simulink model "Channelizer"  (R2026a)
settings: Solver=VariableStepAuto  StopTime=1e-5
InitFcn:
  | init;
values from neighbouring files (symbols this model uses):
  ch0_en = 0    [channelizer_demo_init.m]    (also in init.m)
  ch0_qam = 0    [channelizer_demo_init.m]    (also in init.m)
  ch0_swp = 0    [channelizer_demo_init.m]    (also in init.m)
  ch10_en = 0    [channelizer_demo_init.m]    (also in init.m)
  ch10_qam = 0    [channelizer_demo_init.m]    (also in init.m)
  ch10_swp = 0    [channelizer_demo_init.m]    (also in init.m)
  ch11_en = 0    [channelizer_demo_init.m]    (also in init.m)
  ch11_qam = 0    [channelizer_demo_init.m]    (also in init.m)
  ch11_swp = 0    [channelizer_demo_init.m]    (also in init.m)
  ch12_en = 0    [channelizer_demo_init.m]    (also in init.m)
  ch12_qam = 0    [channelizer_demo_init.m]    (also in init.m)
  ch12_swp = 0    [channelizer_demo_init.m]    (also in init.m)
  ch13_en = 0    [channelizer_demo_init.m]    (also in init.m)
  ch13_qam = 0    [channelizer_demo_init.m]    (also in init.m)
  ch13_swp = 0    [channelizer_demo_init.m]    (also in init.m)
  ch14_en = 0    [channelizer_demo_init.m]    (also in init.m)
  ch14_qam = 0    [channelizer_demo_init.m]    (also in init.m)
  ch14_swp = 0    [channelizer_demo_init.m]    (also in init.m)
  ch15_en = 0    [channelizer_demo_init.m]    (also in init.m)
  ch15_qam = 0    [channelizer_demo_init.m]    (also in init.m)
  ch15_swp = 0    [channelizer_demo_init.m]    (also in init.m)
  ch1_en = 1    [channelizer_demo_init.m]    (also in init.m)
  ch1_qam = 0    [channelizer_demo_init.m]    (also in init.m)
  ch1_swp = 0    [channelizer_demo_init.m]    (also in init.m)
  ch2_en = 1    [channelizer_demo_init.m]    (also in init.m)
  ch2_qam = 0    [channelizer_demo_init.m]    (also in init.m)
  ch2_swp = 0    [channelizer_demo_init.m]    (also in init.m)
  ch3_en = 0    [channelizer_demo_init.m]    (also in init.m)
  ch3_qam = 0    [channelizer_demo_init.m]    (also in init.m)
  ch3_swp = 0    [channelizer_demo_init.m]    (also in init.m)
  ch4_en = 0    [channelizer_demo_init.m]    (also in init.m)
  ch4_qam = 0    [channelizer_demo_init.m]    (also in init.m)
  ch4_swp = 0    [channelizer_demo_init.m]    (also in init.m)
  ch5_en = 1    [channelizer_demo_init.m]    (also in init.m)
  ch5_qam = 1    [channelizer_demo_init.m]    (also in init.m)
  ch5_swp = 0    [channelizer_demo_init.m]    (also in init.m)
  ch6_en = 1    [channelizer_demo_init.m]    (also in init.m)
  ch6_qam = 1    [channelizer_demo_init.m]    (also in init.m)
  ch6_swp = 0    [channelizer_demo_init.m]    (also in init.m)
  ch7_en = 0    [channelizer_demo_init.m]    (also in init.m)
  ch7_qam = 0    [channelizer_demo_init.m]    (also in init.m)
  ch7_swp = 0    [channelizer_demo_init.m]    (also in init.m)
  ch8_en = 0    [channelizer_demo_init.m]    (also in init.m)
  ch8_qam = 0    [channelizer_demo_init.m]    (also in init.m)
  ch8_swp = 0    [channelizer_demo_init.m]    (also in init.m)
  ch9_en = 0    [channelizer_demo_init.m]    (also in init.m)
  ch9_qam = 0    [channelizer_demo_init.m]    (also in init.m)
  ch9_swp = 0    [channelizer_demo_init.m]    (also in init.m)
  ch_filt_coef = 28 * ch_filt_coef / sum(ch_filt_coef(:))    [init.m]
  N = 2*1024    (= 2048)    [hil.m]    (also in init.m = 256)
  nvar = 0.01    [init.m]
  randph = 2*pi*rand(16,1)    [init.m]
  spec1_ch = 1    [channelizer_demo_init.m]    (also in init.m)
  spec2_ch = 2    [channelizer_demo_init.m]    (also in init.m)
  spec3_ch = 5    [channelizer_demo_init.m]    (also in init.m)
  spec4_ch = 6    [channelizer_demo_init.m]    (also in init.m)
  swp_rate0 = 0    [channelizer_demo_init.m]    (also in init.m)
  swp_rate1 = 0    [channelizer_demo_init.m]    (also in init.m)
  swp_rate10 = 0    [channelizer_demo_init.m]    (also in init.m)
  swp_rate11 = 0    [channelizer_demo_init.m]    (also in init.m)
  swp_rate12 = 0    [channelizer_demo_init.m]    (also in init.m)
  swp_rate13 = 0    [channelizer_demo_init.m]    (also in init.m)
  swp_rate14 = 0    [channelizer_demo_init.m]    (also in init.m)
  swp_rate15 = 0    [channelizer_demo_init.m]    (also in init.m)
  swp_rate2 = 0    [channelizer_demo_init.m]    (also in init.m)
  swp_rate3 = 0    [channelizer_demo_init.m]    (also in init.m)
  swp_rate4 = 0    [channelizer_demo_init.m]    (also in init.m)
  swp_rate5 = 0    [channelizer_demo_init.m]    (also in init.m)
  swp_rate6 = 0    [channelizer_demo_init.m]    (also in init.m)
  swp_rate7 = 0    [channelizer_demo_init.m]    (also in init.m)
  swp_rate8 = 0    [channelizer_demo_init.m]    (also in init.m)
  swp_rate9 = 0    [channelizer_demo_init.m]    (also in init.m)
  Ts = 16*(7/4)/8.75e9    (= 3.2e-09)    [init.m]
undefined symbols (not defined in the file or in its folder): Asymmetric, jsin, S, vsva2197, xcvc1902
libraries: aieUtilities x20, aieBasic x7, hlsBasic x4, aieDSP x2, vmcUtilities x1
(part 1 of 3)
settings Model: Creator=robg  LastModifiedBy=robg
settings DebuggingCC: ParameterOverflowMsg=none  ParameterPrecisionLossMsg=none

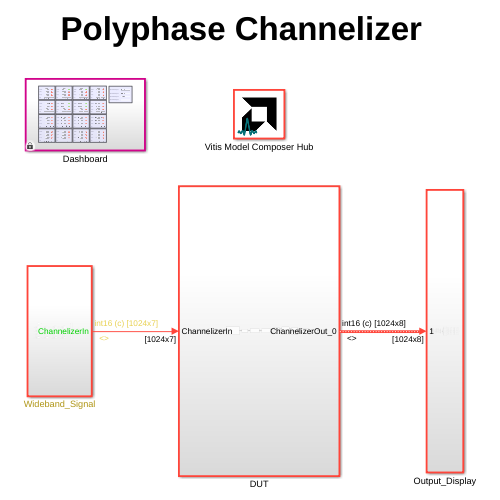
[thumbnail: Simulink's stored preview of the top-level diagram]
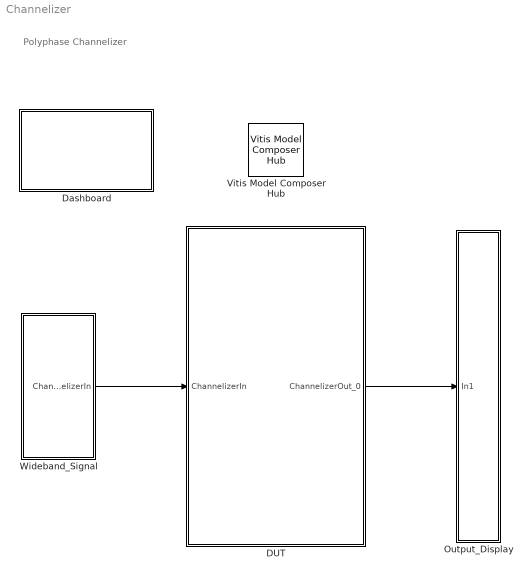
== system Channelizer ==
  note: Polyphase Channelizer
  DUT : Subsystem
  Dashboard : Subsystem
  Output_Display : Subsystem
  Vitis Model Composer Hub : vmcUtilities/Vitis Model Composer Hub  Tag=genX  CodeGeneration=off  SubsystemName=AIE_DFT_SSR  BlockHierPath=Channelizer/DUT/AIE_DFT_SSR  CompilationType=AIECompilation  SubsystemType=AIENode  AIEArrayConfig=Use entire AIE array  StartColumn=1  NumberOfColumns=1  TargetDirectory=./analyze_ssr4  exportDesign=off  analyzeDesign=on  validateDesignOnHw=off  ExportType=AI Engines  IpVendor=xilinx.com  IpLibrary=hls  IpVersion=1.0  IpHWLanguage=Verilog  AieCompilerOptions={}  AieSimulatorOptions={}  CreateTestbench=on  TestbenchStackSize=10  RunRtlSim=off  RunCSim=off  RunAieSim=on  enableSimulationTimeout=on  enableGraphIterations=on  AieSimTimeout=50000  AieGraphIterations=-1  RunAieSimProfiling=on  LaunchVitisAnalyzer=off  PlotOutput=off  RunX86Sim=off  X86SimTimeout=10  GenHwImage=off  GenLibadfXo=off  GenHwValidationCode=off  PlatformType=Not Specified  HwSystemType=Baremetal  HwValidationTarget=hw  ProjDevice=Versal VCK190 Evaluation Platform (xcvc1902-vsva2197-2MP-e-S)  ProjDevicePart=xcvc1902-vsva2197-2MP-e-S  AIEType=AIE  SamplePeriod=-1  ClockFrequency=200  DataPathParallelism=1  xilinxfamily=versalaicore  part=xcvc1902  speed=-2MP-e-S  package=vsva2197  directory=./netlist  testbench=off  incr_netlist=off  synthesis_tool=Vivado  clock_wrapper=Clock Enables  dbl_ovrd=According to Block Masks  dcm_input_clock_period=10  sysclk_period=10  simulink_period=1  eval_field=0  IPInfoJsonString="{\"DUTSubsystemName\":\"AIE_DFT_SSR\",\"AIESubsystem\":{\"SubsystemName\":\"AIE_DFT_SSR\",\"TargetDirectory\":\"./analyze_ssr4\",\"AIEArrayConfig\":\"Use entire AIE array\",\"StartColumn\":\"0\",\"NumberOfColumns\":\"1\"},\"SubsystemTag\":\"AIENode\"}"  LogFileName=/group/xcoswmktg2/robg/git/vmc/Vitis_Model_Composer/Examples/AIENGINE_plus_PL/AIE_HLS/Channelizer/code_dut_ssr_vss/model_composer.log  NThreads=4  IPConfigFile=/tmp/vmctmp-12614866774650903480/Channelizer_ipconfig.json
  Wideband_Signal : Subsystem
  wires:
  DUT/1(ChannelizerOut_0) -> Output_Display/1(In1)
  Wideband_Signal/1(ChannelizerIn) -> DUT/1(ChannelizerIn)

== system Channelizer/DUT ==
  ChannelizerIn : Inport
  AIE to HLS15 : aieUtilities/AIE to HLS  OutputType=ufix128  OutputSize=N  AllowMultiRate=off  InputType=int8
  AIE to HLS16 : aieUtilities/AIE to HLS  OutputType=ufix128  OutputSize=N  AllowMultiRate=off  InputType=int8
  AIE_DFT_SSR : Subsystem
  AIE_FilterBank_SSR : Subsystem
  AIE_to_HLS_IDFT_Out_0 : aieUtilities/AIE to HLS  OutputType=ufix128  OutputSize=1024  AllowMultiRate=off  InputType=cint16
  AIE_to_HLS_IDFT_Out_1 : aieUtilities/AIE to HLS  OutputType=ufix128  OutputSize=1024  AllowMultiRate=off  InputType=cint16
  HLS to AIE17 : aieUtilities/HLS to AIE  OutputType=cint16  OutputSize=4*N  AllowMultiRate=off  InputType=cint16
  HLS_to_AIE_Channel_0 : aieUtilities/HLS to AIE  OutputType=cint16  OutputSize=1024  AllowMultiRate=off  InputType=cint16
  HLS_to_AIE_IDFT_Half0 : aieUtilities/HLS to AIE  OutputType=cint16  OutputSize=2048  AllowMultiRate=off  InputType=cint16
  HLS_to_AIE_IDFT_Half1 : aieUtilities/HLS to AIE  OutputType=cint16  OutputSize=2048  AllowMultiRate=off  InputType=cint16
  idft_output_unpack_kernel : hlsBasic/HLS Kernel  PortNames={'return'; 'half0'; 'half1'; 'hops'}  PortSerializedTypes={'{Bv}';'{C{Thls::stream{2{t{Tap_uint{1{t{}128}}}}{t{}0}}}4}';'{C{Thls::stream{2{t{Tap_uint{1{t{}128}}}}{t{}0}}}4}';'{C{Thls::stream{2{t{Tap_uint{1{t{}128}}}}{t{}0}}}8}'}  FunctionTemplateSpecKind=none  FunctionTemplateParamNames={}  FunctionTemplateParamKinds={}  FunctionTemplateParamTypes={}  FunctionTemplateParamValues={}  PortSynchronicities={'auto'; 'auto'; 'auto'}  PortSignalSizes={0.000000000000000000e+00; 0.000000000000000000e+00; 2.560000000000000000e+02}  PortParameterValues={}  PortAttributesTable={'Input', 'half0', 'hls::stream< ap_uint< 128 >, 0 >[ 4 ]', '', '';'Input', 'half1', 'hls::stream< ap_uint< 128 >, 0 >[ 4 ]', '', '';'Output', 'hops', 'hls::stream< ap_uint< 128 >, 0 >[ 8 ]', '', '256'}  PortAttributesEnablement={'off', 'off', 'off', 'off', 'off';'off', 'off', 'off', 'off', 'off';'off', 'off', 'off', 'off', 'on'}  PortParametersTable={}  SampleTime=-1  PortDirectionTable={'half0', 'hls::stream< ap_uint< 128 >, 0 >[ 4 ]', 'Input', 'Port';'half1', 'hls::stream< ap_uint< 128 >, 0 >[ 4 ]', 'Input', 'Port';'hops', 'hls::stream< ap_uint< 128 >, 0 >[ 8 ]', 'Output', 'Port'}  FunctionTemplateParams={}  FunctionTemplateParamsEnables={}  FunctionTemplateParamsVisible=off  FunctionDeclTypeOptions=C[1 1]@t7@<empty>  PortDirectionTabVisible=on  ArgDirections={1.000000000000000000e+00; 1.000000000000000000e+00; 2.000000000000000000e+00}  ArgInterfaceTypes={1.000000000000000000e+00; 1.000000000000000000e+00; 1.000000000000000000e+00}  FunctionIndex=1  FormalArgDecls={'hls::stream< ap_uint< 128 >, 0 > half0 [ 4 ]';'hls::stream< ap_uint< 128 >, 0 > half1 [ 4 ]';'hls::stream< ap_uint< 128 >, 0 > hops [ 8 ]'}  SimLibPath=''  FunctionTabVisible=on  FunctionDescription=void idft_output_unpack_kernel(hls::stream< ap_uint< 128 >, 0 > half0 [ 4 ], hls::stream< ap_uint< 128 >, 0 > half1 [ 4 ], hls::stream< ap_uint< 128 >, 0 > hops [ 8 ])  blockJsonConstraints=[]  deprecateConstraints=0  KernelHeaderFile=hls/idft_output_unpack_ssr4.h  KernelFunction=idft_output_unpack_kernel  KernelFunctionSelect=<empty>  KernelSourceFile=hls/idft_output_unpack_ssr4.cpp  KernelSearchPaths={}  PreProcOptions={}
  m16_ssr8_cshift_idft_array : hlsBasic/HLS Kernel  PortNames={'return'; 'sig_i'; 'half0'; 'half1'}  PortSerializedTypes={'{Bv}';'{C{Thls::stream{2{t{Tap_uint{1{t{}128}}}}{t{}0}}}8}';'{C{Thls::stream{2{t{Tap_uint{1{t{}128}}}}{t{}0}}}16}';'{C{Thls::stream{2{t{Tap_uint{1{t{}128}}}}{t{}0}}}16}'}  FunctionTemplateSpecKind=none  FunctionTemplateParamNames={}  FunctionTemplateParamKinds={}  FunctionTemplateParamTypes={}  FunctionTemplateParamValues={}  PortSynchronicities={'auto'; 'auto'; 'auto'}  PortSignalSizes={0.000000000000000000e+00; 5.120000000000000000e+02; 5.120000000000000000e+02}  PortParameterValues={}  PortAttributesTable={'Input', 'sig_i', 'hls::stream< ap_uint< 128 >, 0 >[ 8 ]', '', '';'Output', 'half0', 'hls::stream< ap_uint< 128 >, 0 >[ 16 ]', '', '512';'Output', 'half1', 'hls::stream< ap_uint< 128 >, 0 >[ 16 ]', '', '512'}  PortAttributesEnablement={'off', 'off', 'off', 'off', 'off';'off', 'off', 'off', 'off', 'on';'off', 'off', 'off', 'off', 'on'}  PortParametersTable={}  SampleTime=-1  PortDirectionTable={'sig_i', 'hls::stream< ap_uint< 128 >, 0 >[ 8 ]', 'Input', 'Port';'half0', 'hls::stream< ap_uint< 128 >, 0 >[ 16 ]', 'Output', 'Port';'half1', 'hls::stream< ap_uint< 128 >, 0 >[ 16 ]', 'Output', 'Port'}  FunctionTemplateParams={}  FunctionTemplateParamsEnables={}  FunctionTemplateParamsVisible=off  FunctionDeclTypeOptions=C[1 1]@t7@<empty>  PortDirectionTabVisible=on  ArgDirections={1.000000000000000000e+00; 2.000000000000000000e+00; 2.000000000000000000e+00}  ArgInterfaceTypes={1.000000000000000000e+00; 1.000000000000000000e+00; 1.000000000000000000e+00}  FunctionIndex=1  FormalArgDecls={'hls::stream< ap_uint< 128 >, 0 > sig_i [ 8 ]';'hls::stream< ap_uint< 128 >, 0 > half0 [ 16 ]';'hls::stream< ap_uint< 128 >, 0 > half1 [ 16 ]'}  SimLibPath=''  FunctionTabVisible=on  FunctionDescription=void m16_ssr8_cshift_idft_array(hls::stream< ap_uint< 128 >, 0 > sig_i [ 8 ], hls::stream< ap_uint< 128 >, 0 > half0 [ 16 ], hls::stream< ap_uint< 128 >, 0 > half1 [ 16 ])  blockJsonConstraints=[]  deprecateConstraints=0  KernelHeaderFile=hls/m16_ssr8_cyclic_shift_ssr4.h  KernelFunction=m16_ssr8_cshift_idft_array  KernelFunctionSelect=<empty>  KernelSourceFile=hls/m16_ssr8_cyclic_shift_ssr4.cpp  KernelSearchPaths={}  PreProcOptions={}
  m16_ssr8_permute_fb_i_array : hlsBasic/HLS Kernel  PortNames={'return'; 'sig_i'; 'sig_o'}  PortSerializedTypes={'{Bv}'; '{C{Thls::stream{2{t{Tap_uint{1{t{}128}}}}{t{}0}}}7}'; '{C{Thls::stream{2{t{Tap_uint{1{t{}128}}}}{t{}0}}}8}'}  FunctionTemplateSpecKind=none  FunctionTemplateParamNames={}  FunctionTemplateParamKinds={}  FunctionTemplateParamTypes={}  FunctionTemplateParamValues={}  PortSynchronicities={'auto'; 'auto'}  PortSignalSizes={0.000000000000000000e+00; 2.560000000000000000e+02}  PortParameterValues={}  PortAttributesTable={ 'Input', 'sig_i', 'hls::stream< ap_uint< 128 >, 0 >[ 7 ]', '', ''; 'Output', 'sig_o', 'hls::stream< ap_uint< 128 >, 0 >[ 8 ]', '', 'N' }  PortAttributesEnablement={'off', 'off', 'off', 'off', 'off';'off', 'off', 'off', 'off', 'on'}  PortParametersTable={}  SampleTime=-1  PortDirectionTable={ 'sig_i', 'hls::stream< ap_uint< 128 >, 0 >[ 7 ]', 'Input', 'Port'; 'sig_o', 'hls::stream< ap_uint< 128 >, 0 >[ 8 ]', 'Output', 'Port' }  FunctionTemplateParams={}  FunctionTemplateParamsEnables={}  FunctionTemplateParamsVisible=off  FunctionDeclTypeOptions=C[1 1]@t7@<empty>  PortDirectionTabVisible=on  ArgDirections={1.000000000000000000e+00; 2.000000000000000000e+00}  ArgInterfaceTypes={1.000000000000000000e+00; 1.000000000000000000e+00}  FunctionIndex=1  FormalArgDecls={'hls::stream< ap_uint< 128 >, 0 > sig_i [ 7 ]', 'hls::stream< ap_uint< 128 >, 0 > sig_o [ 8 ]'}  SimLibPath=''  FunctionTabVisible=on  FunctionDescription=void m16_ssr8_permute_fb_i_array(hls::stream< ap_uint< 128 >, 0 > sig_i [ 7 ], hls::stream< ap_uint< 128 >, 0 > sig_o [ 8 ])  blockJsonConstraints=[]  deprecateConstraints=0  KernelHeaderFile=hls/m16_ssr8_permute_fb_i.h  KernelFunction=m16_ssr8_permute_fb_i_array  KernelFunctionSelect=<empty>  KernelSourceFile=hls/m16_ssr8_permute_fb_i.cpp  KernelSearchPaths={}  PreProcOptions={}
  m16_ssr8_permute_fb_o_array : hlsBasic/HLS Kernel  PortNames={'return'; 'sig_i'; 'sig_o'}  PortSerializedTypes={'{Bv}'; '{C{Thls::stream{2{t{Tap_uint{1{t{}128}}}}{t{}0}}}8}'; '{C{Thls::stream{2{t{Tap_uint{1{t{}128}}}}{t{}0}}}8}'}  FunctionTemplateSpecKind=none  FunctionTemplateParamNames={}  FunctionTemplateParamKinds={}  FunctionTemplateParamTypes={}  FunctionTemplateParamValues={}  PortSynchronicities={'auto'; 'auto'}  PortSignalSizes={0.000000000000000000e+00; 2.560000000000000000e+02}  PortParameterValues={}  PortAttributesTable={ 'Input', 'sig_i', 'hls::stream< ap_uint< 128 >, 0 >[ 8 ]', '', ''; 'Output', 'sig_o', 'hls::stream< ap_uint< 128 >, 0 >[ 8 ]', '', 'N' }  PortAttributesEnablement={'off', 'off', 'off', 'off', 'off';'off', 'off', 'off', 'off', 'on'}  PortParametersTable={}  SampleTime=-1  PortDirectionTable={ 'sig_i', 'hls::stream< ap_uint< 128 >, 0 >[ 8 ]', 'Input', 'Port'; 'sig_o', 'hls::stream< ap_uint< 128 >, 0 >[ 8 ]', 'Output', 'Port' }  FunctionTemplateParams={}  FunctionTemplateParamsEnables={}  FunctionTemplateParamsVisible=off  FunctionDeclTypeOptions=C[1 1]@t7@<empty>  PortDirectionTabVisible=on  ArgDirections={1.000000000000000000e+00; 2.000000000000000000e+00}  ArgInterfaceTypes={1.000000000000000000e+00; 1.000000000000000000e+00}  FunctionIndex=1  FormalArgDecls={'hls::stream< ap_uint< 128 >, 0 > sig_i [ 8 ]', 'hls::stream< ap_uint< 128 >, 0 > sig_o [ 8 ]'}  SimLibPath=''  FunctionTabVisible=on  FunctionDescription=void m16_ssr8_permute_fb_o_array(hls::stream< ap_uint< 128 >, 0 > sig_i [ 8 ], hls::stream< ap_uint< 128 >, 0 > sig_o [ 8 ])  blockJsonConstraints=[]  deprecateConstraints=0  KernelHeaderFile=hls/m16_ssr8_permute_fb_o.h  KernelFunction=m16_ssr8_permute_fb_o_array  KernelFunctionSelect=<empty>  KernelSourceFile=hls/m16_ssr8_permute_fb_o.cpp  KernelSearchPaths={}  PreProcOptions={}
  ChannelizerOut_0 : Outport
  wires:
  HLS_to_AIE_Channel_0/1 -> ChannelizerOut_0/1
  idft_output_unpack_kernel/1 -> HLS_to_AIE_Channel_0/1
  AIE_to_HLS_IDFT_Out_1/1 -> idft_output_unpack_kernel/2
  ChannelizerIn/1 -> AIE to HLS16/1
  AIE_to_HLS_IDFT_Out_0/1 -> idft_output_unpack_kernel/1
  AIE to HLS16/1 -> m16_ssr8_permute_fb_i_array/1
  AIE_FilterBank_SSR/1(Out1) -> AIE to HLS15/1
  AIE to HLS15/1 -> m16_ssr8_permute_fb_o_array/1
  HLS to AIE17/1 -> AIE_FilterBank_SSR/1(In1)
  HLS_to_AIE_IDFT_Half0/1 -> AIE_DFT_SSR/1(In_Half0)
  m16_ssr8_permute_fb_o_array/1 -> m16_ssr8_cshift_idft_array/1
  m16_ssr8_cshift_idft_array/1 -> HLS_to_AIE_IDFT_Half0/1
  m16_ssr8_cshift_idft_array/2 -> HLS_to_AIE_IDFT_Half1/1
  m16_ssr8_permute_fb_i_array/1 -> HLS to AIE17/1
  HLS_to_AIE_IDFT_Half1/1 -> AIE_DFT_SSR/2(In_Half1)
  AIE_DFT_SSR/1(IDFT_Half0_Out) -> AIE_to_HLS_IDFT_Out_0/1
  AIE_DFT_SSR/2(IDFT_Half1_Out) -> AIE_to_HLS_IDFT_Out_1/1

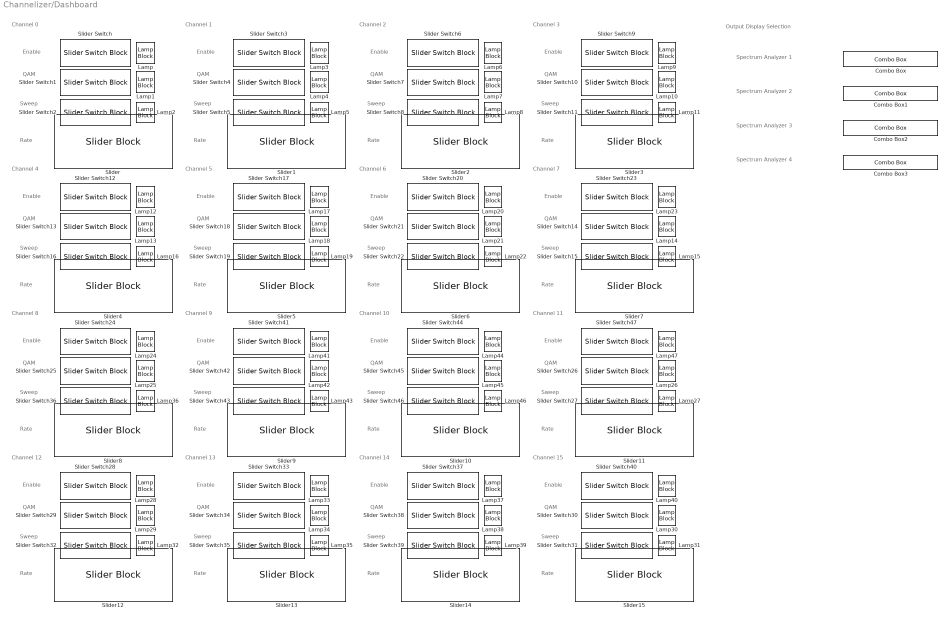
== system Channelizer/Dashboard ==
  note: Output Display Selection
  note: Spectrum Analyzer 1
  note: Enable
  note: Channel 0
  note: QAM
  note: Sweep
  note: Rate
  note: Channel 1
  note: Rate
  note: QAM
  note: Sweep
  note: Enable
  note: Channel 2
  note: Channel 3
  note: Rate
  note: Enable
  note: QAM
  note: Sweep
  note: QAM
  note: Sweep
  note: Rate
  note: Enable
  note: QAM
  note: Enable
  note: Rate
  note: Sweep
  note: Rate
  note: Sweep
  note: Sweep
  note: Channel 5
  note: Channel 6
  note: Rate
  note: Enable
  note: Channel 7
  note: QAM
  note: Sweep
  note: Channel 4
  note: Enable
  note: Enable
  note: QAM
  note: Rate
  note: QAM
  note: Rate
  note: Rate
  note: Sweep
  note: Enable
  note: Rate
  note: Enable
  note: QAM
  note: QAM
  note: Sweep
  note: Channel 11
  note: Sweep
  note: QAM
  note: Rate
  note: Enable
  note: Channel 10
  note: Channel 12
  note: Channel 15
  note: Enable
  note: Enable
  note: Channel 8
  note: QAM
  note: Rate
  note: Sweep
  note: Sweep
  note: QAM
  note: Rate
  note: Channel 14
  note: Enable
  note: QAM
  note: Channel 9
  note: Sweep
  note: QAM
  note: Enable
  note: Sweep
  note: Rate
  note: Sweep
  note: Rate
  note: Channel 13
  note: Enable
  note: QAM
  note: Spectrum Analyzer 2
  note: Spectrum Analyzer 3
  note: Spectrum Analyzer 4
  Combo Box : ComboBox  LabelPosition=Hide  SelectedLabel=Channel 1
  Combo Box1 : ComboBox  LabelPosition=Hide  SelectedLabel=Channel 2
  Combo Box2 : ComboBox  LabelPosition=Hide  SelectedLabel=Channel 5
  Combo Box3 : ComboBox  LabelPosition=Hide  SelectedLabel=Channel 6
  Lamp{,1..47} (48 alike) : LampBlock  LabelPosition=Hide  DefaultColor=[192.0, 192.0, 192.0]
  Slider{,1..15} (16 alike) : SliderBlock  LabelPosition=Hide  ScaleMin=-1  ScaleMax=1
  Slider Switch{,1..47} (48 alike) : SliderSwitchBlock  LabelPosition=Hide

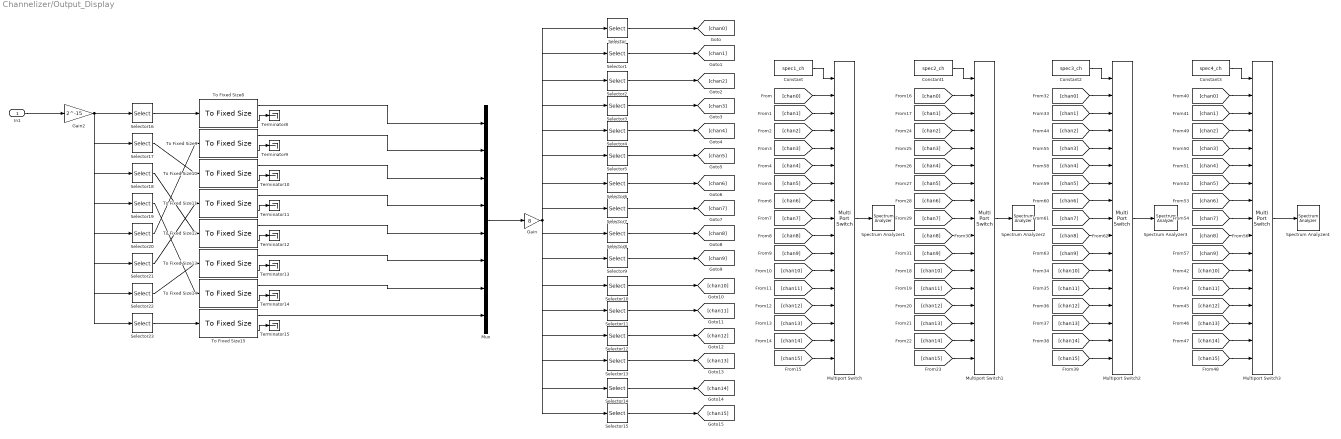
== system Channelizer/Output_Display ==
  In1 : Inport
  Constant : Constant  Value=spec1_ch  SampleTime=-1
  Constant1 : Constant  Value=spec2_ch  SampleTime=-1
  Constant2 : Constant  Value=spec3_ch  SampleTime=-1
  Constant3 : Constant  Value=spec4_ch  SampleTime=-1
  Gain : Gain  Gain=8
  Gain2 : Gain  Gain=2^-15  OutDataTypeStr=double
  Multiport Switch{,1..3} (4 alike) : MultiPortSwitch  DataPortOrder=Zero-based contiguous  Inputs=16  zeroidx=on  SaturateOnIntegerOverflow=off  InputSameDT=off
  Mux : Mux  Inputs=8
  Selector : Selector  InputPortWidth=32*N  IndexOptions=Index vector (dialog)  Indices=reshape([(1:4:(4*N))' ((4*N+1):4:(8*N))']',2*N,1)  OutputSizes=1
  Selector1 : Selector  InputPortWidth=32*N  IndexOptions=Index vector (dialog)  Indices=reshape([(2:4:(4*N))' ((4*N+2):4:(8*N))']',2*N,1)  OutputSizes=1
  Selector10 : Selector  InputPortWidth=32*N  IndexOptions=Index vector (dialog)  Indices=reshape([((16*N+3):4:(20*N))' ((20*N+3):4:(24*N))']',2*N,1)  OutputSizes=1
  Selector11 : Selector  InputPortWidth=32*N  IndexOptions=Index vector (dialog)  Indices=reshape([((16*N+4):4:(20*N))' ((20*N+4):4:(24*N))']',2*N,1)  OutputSizes=1
  Selector12 : Selector  InputPortWidth=32*N  IndexOptions=Index vector (dialog)  Indices=reshape([((24*N+1):4:(28*N))' ((28*N+1):4:(32*N))']',2*N,1)  OutputSizes=1
  Selector13 : Selector  InputPortWidth=32*N  IndexOptions=Index vector (dialog)  Indices=reshape([((24*N+2):4:(28*N))' ((28*N+2):4:(32*N))']',2*N,1)  OutputSizes=1
  Selector14 : Selector  InputPortWidth=32*N  IndexOptions=Index vector (dialog)  Indices=reshape([((24*N+3):4:(28*N))' ((28*N+3):4:(32*N))']',2*N,1)  OutputSizes=1
  Selector15 : Selector  InputPortWidth=32*N  IndexOptions=Index vector (dialog)  Indices=reshape([((24*N+4):4:(28*N))' ((28*N+4):4:(32*N))']',2*N,1)  OutputSizes=1
  Selector16 : Selector  NumberOfDimensions=2  InputPortWidth=3  IndexOptions=Select all,Index vector (dialog)  Indices=,1  OutputSizes=1,1
  Selector17 : Selector  NumberOfDimensions=2  InputPortWidth=3  IndexOptions=Select all,Index vector (dialog)  Indices=,3  OutputSizes=1,1
  Selector18 : Selector  NumberOfDimensions=2  InputPortWidth=3  IndexOptions=Select all,Index vector (dialog)  Indices=,5  OutputSizes=1,1
  Selector19 : Selector  NumberOfDimensions=2  InputPortWidth=3  IndexOptions=Select all,Index vector (dialog)  Indices=,7  OutputSizes=1,1
  Selector2 : Selector  InputPortWidth=32*N  IndexOptions=Index vector (dialog)  Indices=reshape([(3:4:(4*N))' ((4*N+3):4:(8*N))']',2*N,1)  OutputSizes=1
  Selector20 : Selector  NumberOfDimensions=2  InputPortWidth=3  IndexOptions=Select all,Index vector (dialog)  Indices=,2  OutputSizes=1,1
  Selector21 : Selector  NumberOfDimensions=2  InputPortWidth=3  IndexOptions=Select all,Index vector (dialog)  Indices=,4  OutputSizes=1,1
  Selector22 : Selector  NumberOfDimensions=2  InputPortWidth=3  IndexOptions=Select all,Index vector (dialog)  Indices=,6  OutputSizes=1,1
  Selector23 : Selector  NumberOfDimensions=2  InputPortWidth=3  IndexOptions=Select all,Index vector (dialog)  Indices=,8  OutputSizes=1,1
  Selector3 : Selector  InputPortWidth=32*N  IndexOptions=Index vector (dialog)  Indices=reshape([(4:4:(4*N))' ((4*N+4):4:(8*N))']',2*N,1)  OutputSizes=1
  Selector4 : Selector  InputPortWidth=32*N  IndexOptions=Index vector (dialog)  Indices=reshape([((8*N+1):4:(12*N))' ((12*N+1):4:(16*N))']',2*N,1)  OutputSizes=1
  Selector5 : Selector  InputPortWidth=32*N  IndexOptions=Index vector (dialog)  Indices=reshape([((8*N+2):4:(12*N))' ((12*N+2):4:(16*N))']',2*N,1)  OutputSizes=1
  Selector6 : Selector  InputPortWidth=32*N  IndexOptions=Index vector (dialog)  Indices=reshape([((8*N+3):4:(12*N))' ((12*N+3):4:(16*N))']',2*N,1)  OutputSizes=1
  Selector7 : Selector  InputPortWidth=32*N  IndexOptions=Index vector (dialog)  Indices=reshape([((8*N+4):4:(12*N))' ((12*N+4):4:(16*N))']',2*N,1)  OutputSizes=1
  Selector8 : Selector  InputPortWidth=32*N  IndexOptions=Index vector (dialog)  Indices=reshape([((16*N+1):4:(20*N))' ((20*N+1):4:(24*N))']',2*N,1)  OutputSizes=1
  Selector9 : Selector  InputPortWidth=32*N  IndexOptions=Index vector (dialog)  Indices=reshape([((16*N+2):4:(20*N))' ((20*N+2):4:(24*N))']',2*N,1)  OutputSizes=1
  Spectrum Analyzer1 : SpectrumAnalyzer  WindowPosition=[74.000000,541.000000,568.000000,295.000000,]  Visible=on  ScopeFrameLocation=window  AxesScaling=Manual  Span=625000000  StartFrequency=-312500000  StopFrequency=312500000  AveragingMethod=Exponential  YLimits=[-41.57354089,34.98021919]  ChannelNames="[\"\"]"  AllowFFTLengthLessThanSamplesPerUpdate=on  DefaultConfigurationName=spbscopes.SpectrumAnalyzerBlockCfg
  Spectrum Analyzer2 : SpectrumAnalyzer  WindowPosition=[688.000000,478.000000,567.000000,285.000000,]  Visible=on  ScopeFrameLocation=window  AxesScaling=Manual  Span=625000000  StartFrequency=-312500000  StopFrequency=312500000  AveragingMethod=Exponential  YLimits=[-43.59374281,36.64610385]  ChannelNames="[\"\"]"  AllowFFTLengthLessThanSamplesPerUpdate=on  DefaultConfigurationName=spbscopes.SpectrumAnalyzerBlockCfg
  Spectrum Analyzer3 : SpectrumAnalyzer  WindowPosition=[1181.000000,128.000000,569.000000,310.000000,]  Visible=on  ScopeFrameLocation=window  AxesScaling=Manual  Span=625000000  StartFrequency=-312500000  StopFrequency=312500000  AveragingMethod=Exponential  ChannelNames="[\"\"]"  AllowFFTLengthLessThanSamplesPerUpdate=on  DefaultConfigurationName=spbscopes.SpectrumAnalyzerBlockCfg
  Spectrum Analyzer4 : SpectrumAnalyzer  WindowPosition=[50.000000,76.000000,574.000000,367.000000,]  Visible=on  ScopeFrameLocation=window  AxesScaling=Manual  Span=625000000  StartFrequency=-312500000  StopFrequency=312500000  AveragingMethod=Exponential  ChannelNames="[\"\"]"  AllowFFTLengthLessThanSamplesPerUpdate=on  DefaultConfigurationName=spbscopes.SpectrumAnalyzerBlockCfg
  Terminator{8..15} (8 alike) : Terminator
  To Fixed Size{8..15} (8 alike) : aieUtilities/To Fixed Size  Mode=Produce a valid output signal  OutputSize=Inherit: Same as input  CopyMethod=Buffer samples to form output  HasStatusOutput=on
  wires:
  [chan15] -> Multiport Switch/17
  [chan14] -> Multiport Switch/16
  [chan13] -> Multiport Switch/15
  [chan12] -> Multiport Switch/14
  [chan11] -> Multiport Switch/13
  [chan4] -> Multiport Switch/6
  [chan5] -> Multiport Switch/7
  [chan6] -> Multiport Switch/8
  [chan7] -> Multiport Switch/9
  [chan10] -> Multiport Switch/12
  [chan9] -> Multiport Switch/11
  [chan8] -> Multiport Switch/10
  [chan3] -> Multiport Switch/5
  [chan2] -> Multiport Switch/4
  [chan1] -> Multiport Switch/3
  [chan0] -> Multiport Switch/2
  Multiport Switch/1 -> Spectrum Analyzer1/1
  Constant/1 -> Multiport Switch/1
  [chan1] -> Multiport Switch1/3
  [chan15] -> Multiport Switch1/17
  [chan5] -> Multiport Switch1/7
  [chan14] -> Multiport Switch1/16
  [chan3] -> Multiport Switch1/5
  [chan2] -> Multiport Switch1/4
  [chan6] -> Multiport Switch1/8
  [chan7] -> Multiport Switch1/9
  [chan12] -> Multiport Switch1/14
  Multiport Switch1/1 -> Spectrum Analyzer2/1
  [chan0] -> Multiport Switch1/2
  [chan4] -> Multiport Switch1/6
  [chan9] -> Multiport Switch1/11
  [chan10] -> Multiport Switch1/12
  [chan8] -> Multiport Switch1/10
  [chan11] -> Multiport Switch1/13
  Constant1/1 -> Multiport Switch1/1
  [chan13] -> Multiport Switch1/15
  [chan1] -> Multiport Switch3/3
  [chan8] -> Multiport Switch3/10
  [chan8] -> Multiport Switch2/10
  [chan4] -> Multiport Switch3/6
  Multiport Switch3/1 -> Spectrum Analyzer4/1
  [chan0] -> Multiport Switch2/2
  [chan14] -> Multiport Switch2/16
  [chan3] -> Multiport Switch2/5
  [chan9] -> Multiport Switch3/11
  [chan0] -> Multiport Switch3/2
  [chan15] -> Multiport Switch2/17
  [chan10] -> Multiport Switch3/12
  [chan9] -> Multiport Switch2/11
  [chan6] -> Multiport Switch2/8
  Constant3/1 -> Multiport Switch3/1
  [chan1] -> Multiport Switch2/3
  [chan7] -> Multiport Switch2/9
  [chan14] -> Multiport Switch3/16
  [chan4] -> Multiport Switch2/6
  [chan7] -> Multiport Switch3/9
  [chan15] -> Multiport Switch3/17
  [chan10] -> Multiport Switch2/12
  [chan3] -> Multiport Switch3/5
  [chan13] -> Multiport Switch3/15
  Constant2/1 -> Multiport Switch2/1
  [chan5] -> Multiport Switch3/7
  [chan5] -> Multiport Switch2/7
  Multiport Switch2/1 -> Spectrum Analyzer3/1
  [chan12] -> Multiport Switch2/14
  [chan2] -> Multiport Switch2/4
  [chan2] -> Multiport Switch3/4
  [chan6] -> Multiport Switch3/8
  [chan11] -> Multiport Switch2/13
  [chan13] -> Multiport Switch2/15
  [chan11] -> Multiport Switch3/13
  [chan12] -> Multiport Switch3/14
  To Fixed Size8/2 -> Terminator8/1
  To Fixed Size9/2 -> Terminator9/1
  To Fixed Size10/2 -> Terminator10/1
  To Fixed Size11/2 -> Terminator11/1
  To Fixed Size12/2 -> Terminator12/1
  To Fixed Size13/2 -> Terminator13/1
  To Fixed Size14/2 -> Terminator14/1
  To Fixed Size15/2 -> Terminator15/1
  Mux/1 -> Gain/1
  Selector/1 -> [chan0]
  Selector1/1 -> [chan1]
  Selector2/1 -> [chan2]
  Selector3/1 -> [chan3]
  Selector4/1 -> [chan4]
  Selector5/1 -> [chan5]
  Selector6/1 -> [chan6]
  Selector7/1 -> [chan7]
  Selector8/1 -> [chan8]
  Selector9/1 -> [chan9]
  Selector10/1 -> [chan10]
  Selector11/1 -> [chan11]
  Selector12/1 -> [chan12]
  Selector13/1 -> [chan13]
  Selector14/1 -> [chan14]
  Selector15/1 -> [chan15]
  To Fixed Size8/1 -> Mux/1
  To Fixed Size9/1 -> Mux/2
  To Fixed Size10/1 -> Mux/3
  To Fixed Size11/1 -> Mux/4
  To Fixed Size12/1 -> Mux/5
  To Fixed Size13/1 -> Mux/6
  To Fixed Size14/1 -> Mux/7
  To Fixed Size15/1 -> Mux/8
  In1/1 -> Gain2/1
  Selector16/1 -> To Fixed Size8/1
  Selector17/1 -> To Fixed Size10/1
  Selector18/1 -> To Fixed Size12/1
  Selector19/1 -> To Fixed Size14/1
  Selector20/1 -> To Fixed Size9/1
  Selector21/1 -> To Fixed Size11/1
  Selector22/1 -> To Fixed Size13/1
  Selector23/1 -> To Fixed Size15/1
  Gain2/1 -> Selector16/1, Selector17/1, Selector18/1, Selector19/1, Selector20/1, Selector21/1, Selector22/1, Selector23/1
  Gain/1 -> Selector/1, Selector1/1, Selector2/1, Selector3/1, Selector4/1, Selector5/1, Selector6/1, Selector7/1, Selector8/1, Selector9/1, Selector10/1, Selector11/1, Selector12/1, Selector13/1, Selector14/1, Selector15/1

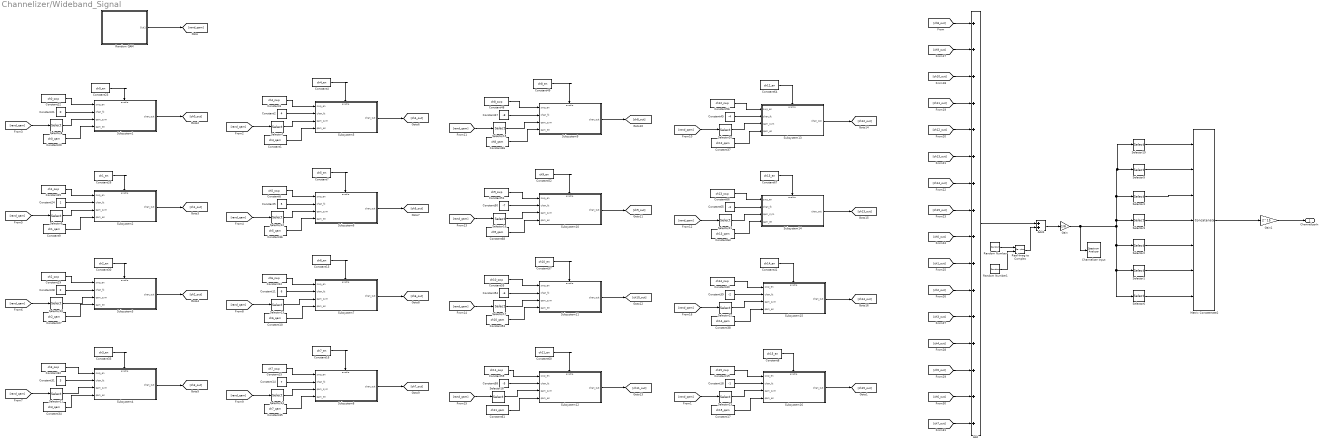
== system Channelizer/Wideband_Signal ==
  Add : Sum  Inputs=++++++++++++++++
  Add1 : Sum
  Channelizer Input : SpectrumAnalyzer  WindowPosition=[557.000000,65.000000,800.000000,381.000000,]  Visible=on  ScopeFrameLocation=window  Span=8750000000  StartFrequency=-4375000000  StopFrequency=4375000000  AveragingMethod=Running  ForgettingFactor=0.4  YLimits=[-73.2173 24.2048]  ChannelNames="[\"\"]"  AllowFFTLengthLessThanSamplesPerUpdate=on  DefaultConfigurationName=spbscopes.SpectrumAnalyzerBlockCfg
  Constant1 : Constant  Value=ch4_qam  SampleTime=-1
  Constant10 : Constant  Value=ch6_qam  SampleTime=-1
  Constant11 : Constant  Value=6  SampleTime=-1
  Constant12 : Constant  Value=ch6_swp  SampleTime=-1
  Constant13 : Constant  Value=ch6_en  SampleTime=-1
  Constant14 : Constant  Value=7  SampleTime=-1
  Constant15 : Constant  Value=ch7_swp  SampleTime=-1
  Constant16 : Constant  Value=ch7_en  SampleTime=-1
  Constant17 : Constant  Value=ch15_qam  SampleTime=-1
  Constant18 : Constant  Value=-1  SampleTime=-1
  Constant19 : Constant  Value=ch15_swp  SampleTime=-1
  Constant2 : Constant  Value=4  SampleTime=-1
  Constant20 : Constant  Value=ch0_qam  SampleTime=-1
  Constant21 : Constant  Value=0  SampleTime=-1
  Constant22 : Constant  Value=ch0_swp  SampleTime=-1
  Constant23 : Constant  Value=ch0_en  SampleTime=-1
  Constant24 : Constant  SampleTime=-1
  Constant25 : Constant  Value=ch1_swp  SampleTime=-1
  Constant26 : Constant  Value=ch1_en  SampleTime=-1
  Constant27 : Constant  Value=ch2_qam  SampleTime=-1
  Constant28 : Constant  Value=2  SampleTime=-1
  Constant29 : Constant  Value=ch2_swp  SampleTime=-1
  Constant3 : Constant  Value=ch4_swp  SampleTime=-1
  Constant30 : Constant  Value=ch2_en  SampleTime=-1
  Constant31 : Constant  Value=3  SampleTime=-1
  Constant32 : Constant  Value=ch3_swp  SampleTime=-1
  Constant33 : Constant  Value=ch3_en  SampleTime=-1
  Constant34 : Constant  Value=ch3_qam  SampleTime=-1
  Constant35 : Constant  Value=ch7_qam  SampleTime=-1
  Constant36 : Constant  Value=ch5_qam  SampleTime=-1
  Constant37 : Constant  Value=ch12_qam  SampleTime=-1
  Constant38 : Constant  Value=ch14_qam  SampleTime=-1
  Constant39 : Constant  Value=-2  SampleTime=-1
  Constant4 : Constant  Value=ch4_en  SampleTime=-1
  Constant40 : Constant  Value=ch14_swp  SampleTime=-1
  Constant41 : Constant  Value=ch14_en  SampleTime=-1
  Constant45 : Constant  Value=-4  SampleTime=-1
  Constant46 : Constant  Value=ch8_qam  SampleTime=-1
  Constant47 : Constant  Value=-8  SampleTime=-1
  Constant48 : Constant  Value=ch8_swp  SampleTime=-1
  Constant49 : Constant  Value=ch8_en  SampleTime=-1
  Constant5 : Constant  Value=5  SampleTime=-1
  Constant50 : Constant  Value=-7  SampleTime=-1
  Constant51 : Constant  Value=ch9_swp  SampleTime=-1
  Constant52 : Constant  Value=ch9_en  SampleTime=-1
  Constant53 : Constant  Value=ch10_qam  SampleTime=-1
  Constant54 : Constant  Value=-6  SampleTime=-1
  Constant55 : Constant  Value=ch10_swp  SampleTime=-1
  Constant56 : Constant  Value=ch12_swp  SampleTime=-1
  Constant57 : Constant  Value=ch10_en  SampleTime=-1
  Constant58 : Constant  Value=-5  SampleTime=-1
  Constant59 : Constant  Value=ch11_swp  SampleTime=-1
  Constant6 : Constant  Value=ch5_swp  SampleTime=-1
  Constant60 : Constant  Value=ch11_en  SampleTime=-1
  Constant61 : Constant  Value=ch11_qam  SampleTime=-1
  Constant63 : Constant  Value=ch13_qam  SampleTime=-1
  Constant64 : Constant  Value=ch12_en  SampleTime=-1
  Constant65 : Constant  Value=-3  SampleTime=-1
  Constant66 : Constant  Value=ch13_swp  SampleTime=-1
  Constant67 : Constant  Value=ch13_en  SampleTime=-1
  Constant68 : Constant  Value=ch9_qam  SampleTime=-1
  Constant7 : Constant  Value=ch5_en  SampleTime=-1
  Constant8 : Constant  Value=ch15_en  SampleTime=-1
  Constant9 : Constant  Value=ch1_qam  SampleTime=-1
  Gain : Gain  Gain=1/6
  Gain1 : Gain  Gain=2^15  OutDataTypeStr=int16
  Matrix Concatenate2 : Concatenate  NumInputs=7  Mode=Multidimensional array  ConcatenateDimension=2
  Random Number : RandomNumber  Variance=nvar  Seed=1234*(1:28*N)'  SampleTime=Ts*N  VectorParams1D=off
  Random Number1 : RandomNumber  Variance=nvar  Seed=543*(1:28*N)'  SampleTime=Ts*N  VectorParams1D=off
  Random QAM : Subsystem
  Real-Imag to Complex : RealImagToComplex
  Selector1 : Selector  InputPortWidth=28*N  IndexOptions=Index vector (dialog)  Indices=reshape([(9:14:28*N)' (2:14:28*N)']',4*N,1)  OutputSizes=1
  Selector10 : Selector  InputPortWidth=16*N  IndexOptions=Index vector (dialog)  Indices=3:16:16*N  OutputSizes=1
  Selector11 : Selector  InputPortWidth=16*N  IndexOptions=Index vector (dialog)  Indices=4:16:16*N  OutputSizes=1
  Selector12 : Selector  InputPortWidth=16*N  IndexOptions=Index vector (dialog)  Indices=6:16:16*N  OutputSizes=1
  Selector13 : Selector  InputPortWidth=16*N  IndexOptions=Index vector (dialog)  Indices=7:16:16*N  OutputSizes=1
  Selector14 : Selector  InputPortWidth=16*N  IndexOptions=Index vector (dialog)  Indices=8:16:16*N  OutputSizes=1
  Selector15 : Selector  InputPortWidth=16*N  IndexOptions=Index vector (dialog)  Indices=9:16:16*N  OutputSizes=1
  Selector16 : Selector  InputPortWidth=16*N  IndexOptions=Index vector (dialog)  Indices=10:16:16*N  OutputSizes=1
  Selector17 : Selector  InputPortWidth=16*N  IndexOptions=Index vector (dialog)  Indices=11:16:16*N  OutputSizes=1
  Selector18 : Selector  InputPortWidth=16*N  IndexOptions=Index vector (dialog)  Indices=12:16:16*N  OutputSizes=1
  Selector19 : Selector  InputPortWidth=28*N  IndexOptions=Index vector (dialog)  Indices=reshape([(14:14:28*N)' (7:14:28*N)']',4*N,1)  OutputSizes=1
  Selector2 : Selector  InputPortWidth=28*N  IndexOptions=Index vector (dialog)  Indices=reshape([(10:14:28*N)' (3:14:28*N)']',4*N,1)  OutputSizes=1
  Selector20 : Selector  InputPortWidth=16*N  IndexOptions=Index vector (dialog)  Indices=13:16:16*N  OutputSizes=1
  Selector21 : Selector  InputPortWidth=16*N  IndexOptions=Index vector (dialog)  Indices=14:16:16*N  OutputSizes=1
  Selector22 : Selector  InputPortWidth=16*N  IndexOptions=Index vector (dialog)  Indices=15:16:16*N  OutputSizes=1
  Selector23 : Selector  InputPortWidth=16*N  IndexOptions=Index vector (dialog)  Indices=16:16:16*N  OutputSizes=1
  Selector3 : Selector  InputPortWidth=28*N  IndexOptions=Index vector (dialog)  Indices=reshape([(11:14:28*N)' (4:14:28*N)']',4*N,1)  OutputSizes=1
  Selector4 : Selector  InputPortWidth=28*N  IndexOptions=Index vector (dialog)  Indices=reshape([(12:14:28*N)' (5:14:28*N)']',4*N,1)  OutputSizes=1
  Selector5 : Selector  InputPortWidth=28*N  IndexOptions=Index vector (dialog)  Indices=reshape([(13:14:28*N)' (6:14:28*N)']',4*N,1)  OutputSizes=1
  Selector6 : Selector  InputPortWidth=28*N  IndexOptions=Index vector (dialog)  Indices=reshape([(8:14:28*N)' (1:14:28*N)']',4*N,1)  OutputSizes=1
  Selector7 : Selector  InputPortWidth=16*N  IndexOptions=Index vector (dialog)  Indices=5:16:16*N  OutputSizes=1
  Selector8 : Selector  InputPortWidth=16*N  IndexOptions=Index vector (dialog)  Indices=1:16:16*N  OutputSizes=1
  Selector9 : Selector  InputPortWidth=16*N  IndexOptions=Index vector (dialog)  Indices=2:16:16*N  OutputSizes=1
  Subsystem1 : Subsystem
  Subsystem10 : Subsystem
  Subsystem11 : Subsystem
  Subsystem12 : Subsystem
  Subsystem13 : Subsystem
  Subsystem14 : Subsystem
  Subsystem15 : Subsystem
  Subsystem16 : Subsystem
  Subsystem2 : Subsystem
  Subsystem3 : Subsystem
  Subsystem4 : Subsystem
  Subsystem5 : Subsystem
  Subsystem6 : Subsystem
  Subsystem7 : Subsystem
  Subsystem8 : Subsystem
  Subsystem9 : Subsystem
  ChannelizerIn : Outport
  wires:
  Constant18/1 -> Subsystem16/2(chan_fc)
  Constant19/1 -> Subsystem16/1(swp_en)
  Constant8/1 -> Subsystem16/Enable
  Constant17/1 -> Subsystem16/4(qam_en)
  Selector23/1 -> Subsystem16/3(qam_sym)
  [rand_qam] -> Selector23/1
  Subsystem16/1(chan_out) -> [ch15_out]
  Constant20/1 -> Subsystem1/4(qam_en)
  Selector8/1 -> Subsystem1/3(qam_sym)
  Constant23/1 -> Subsystem1/Enable
  Constant21/1 -> Subsystem1/2(chan_fc)
  Constant22/1 -> Subsystem1/1(swp_en)
  Subsystem2/1(chan_out) -> [ch1_out]
  Selector9/1 -> Subsystem2/3(qam_sym)
  [rand_qam] -> Selector9/1
  Constant26/1 -> Subsystem2/Enable
  Constant24/1 -> Subsystem2/2(chan_fc)
  Constant9/1 -> Subsystem2/4(qam_en)
  Constant25/1 -> Subsystem2/1(swp_en)
  [rand_qam] -> Selector11/1
  Constant28/1 -> Subsystem3/2(chan_fc)
  Constant29/1 -> Subsystem3/1(swp_en)
  Selector11/1 -> Subsystem4/3(qam_sym)
  Constant32/1 -> Subsystem4/1(swp_en)
  Constant30/1 -> Subsystem3/Enable
  [rand_qam] -> Selector10/1
  Selector10/1 -> Subsystem3/3(qam_sym)
  Subsystem4/1(chan_out) -> [ch3_out]
  Constant33/1 -> Subsystem4/Enable
  Constant31/1 -> Subsystem4/2(chan_fc)
  Constant27/1 -> Subsystem3/4(qam_en)
  Subsystem3/1(chan_out) -> [ch2_out]
  Constant34/1 -> Subsystem4/4(qam_en)
  Constant2/1 -> Subsystem5/2(chan_fc)
  [rand_qam] -> Selector12/1
  Constant12/1 -> Subsystem7/1(swp_en)
  Constant15/1 -> Subsystem8/1(swp_en)
  Constant5/1 -> Subsystem6/2(chan_fc)
  Constant35/1 -> Subsystem8/4(qam_en)
  Constant36/1 -> Subsystem6/4(qam_en)
  [rand_qam] -> Selector14/1
  Selector7/1 -> Subsystem5/3(qam_sym)
  Subsystem6/1(chan_out) -> [ch5_out]
  Constant7/1 -> Subsystem6/Enable
  Subsystem8/1(chan_out) -> [ch7_out]
  Subsystem5/1(chan_out) -> [ch4_out]
  Constant4/1 -> Subsystem5/Enable
  Constant16/1 -> Subsystem8/Enable
  Constant1/1 -> Subsystem5/4(qam_en)
  Subsystem7/1(chan_out) -> [ch6_out]
  Constant13/1 -> Subsystem7/Enable
  Constant6/1 -> Subsystem6/1(swp_en)
  [rand_qam] -> Selector7/1
  Selector12/1 -> Subsystem6/3(qam_sym)
  Constant3/1 -> Subsystem5/1(swp_en)
  Selector14/1 -> Subsystem8/3(qam_sym)
  [rand_qam] -> Selector13/1
  Constant14/1 -> Subsystem8/2(chan_fc)
  Subsystem9/1(chan_out) -> [ch8_out]
  Selector20/1 -> Subsystem13/3(qam_sym)
  Constant68/1 -> Subsystem10/4(qam_en)
  Constant47/1 -> Subsystem9/2(chan_fc)
  Constant37/1 -> Subsystem13/4(qam_en)
  Selector17/1 -> Subsystem11/3(qam_sym)
  Constant63/1 -> Subsystem14/4(qam_en)
  Constant56/1 -> Subsystem13/1(swp_en)
  Selector15/1 -> Subsystem9/3(qam_sym)
  [rand_qam] -> Selector21/1
  [rand_qam] -> Selector20/1
  Constant61/1 -> Subsystem12/4(qam_en)
  Constant39/1 -> Subsystem15/2(chan_fc)
  Subsystem14/1(chan_out) -> [ch13_out]
  Constant60/1 -> Subsystem12/Enable
  Constant66/1 -> Subsystem14/1(swp_en)
  Constant51/1 -> Subsystem10/1(swp_en)
  Constant67/1 -> Subsystem14/Enable
  Constant49/1 -> Subsystem9/Enable
  Constant65/1 -> Subsystem14/2(chan_fc)
  Subsystem11/1(chan_out) -> [ch10_out]
  [rand_qam] -> Selector22/1
  Selector16/1 -> Subsystem10/3(qam_sym)
  Constant55/1 -> Subsystem11/1(swp_en)
  Constant59/1 -> Subsystem12/1(swp_en)
  Constant52/1 -> Subsystem10/Enable
  Constant45/1 -> Subsystem13/2(chan_fc)
  Constant40/1 -> Subsystem15/1(swp_en)
  Subsystem10/1(chan_out) -> [ch9_out]
  Subsystem13/1(chan_out) -> [ch12_out]
  Selector22/1 -> Subsystem15/3(qam_sym)
  Constant64/1 -> Subsystem13/Enable
  Selector18/1 -> Subsystem12/3(qam_sym)
  Constant53/1 -> Subsystem11/4(qam_en)
  [rand_qam] -> Selector18/1
  Constant46/1 -> Subsystem9/4(qam_en)
  Selector21/1 -> Subsystem14/3(qam_sym)
  Constant57/1 -> Subsystem11/Enable
  [rand_qam] -> Selector15/1
  Subsystem15/1(chan_out) -> [ch14_out]
  Constant54/1 -> Subsystem11/2(chan_fc)
  Constant41/1 -> Subsystem15/Enable
  Constant48/1 -> Subsystem9/1(swp_en)
  Constant50/1 -> Subsystem10/2(chan_fc)
  [rand_qam] -> Selector17/1
  Constant58/1 -> Subsystem12/2(chan_fc)
  Constant38/1 -> Subsystem15/4(qam_en)
  Subsystem12/1(chan_out) -> [ch11_out]
  [rand_qam] -> Selector16/1
  Add1/1 -> Gain/1
  Gain/1 -> Selector3/1, Selector4/1, Selector5/1, Selector19/1, Selector1/1, Selector6/1, Selector2/1, Channelizer Input/1
  Constant10/1 -> Subsystem7/4(qam_en)
  Selector13/1 -> Subsystem7/3(qam_sym)
  Constant11/1 -> Subsystem7/2(chan_fc)
  Gain1/1 -> ChannelizerIn/1
  Add/1 -> Add1/1
  Subsystem1/1(chan_out) -> [ch0_out]
  [rand_qam] -> Selector8/1
  Random QAM/1(Out1) -> [rand_qam]
  [ch0_out] -> Add/9
  [ch1_out] -> Add/10
  [ch2_out] -> Add/11
  [ch3_out] -> Add/12
  [ch4_out] -> Add/13
  [ch5_out] -> Add/14
  [ch6_out] -> Add/15
  [ch7_out] -> Add/16
  [ch8_out] -> Add/1
  [ch9_out] -> Add/2
  [ch10_out] -> Add/3
  [ch11_out] -> Add/4
  [ch12_out] -> Add/5
  [ch13_out] -> Add/6
  [ch14_out] -> Add/7
  [ch15_out] -> Add/8
  Random Number/1 -> Real-Imag to Complex/1
  Random Number1/1 -> Real-Imag to Complex/2
  Real-Imag to Complex/1 -> Add1/2
  Matrix Concatenate2/1 -> Gain1/1
  Selector19/1 -> Matrix Concatenate2/1
  Selector5/1 -> Matrix Concatenate2/2
  Selector4/1 -> Matrix Concatenate2/3
  Selector3/1 -> Matrix Concatenate2/4
  Selector2/1 -> Matrix Concatenate2/5
  Selector1/1 -> Matrix Concatenate2/6
  Selector6/1 -> Matrix Concatenate2/7

== system Channelizer/DUT/AIE_DFT_SSR ==
  In_Half0 : Inport
  In_Half1 : Inport  Port=2
  IDFT_Half0 : aieDSP/IDFT  data_type=cint16  twiddle_type=cint16  point_size=16  num_frames=256  shift_val=0  rnd_mode=Round to positive infinity  ssr=4  sat_mode=1-Asymmetric  casc_length=4  AIE_VARIANT=1  TP_API=0  TP_FFT_NIFFT=0  blockJsonConstraints=[]  blockJsonConstraintsInternal=[]  spec=vmc_idft.json  SerializedMaskParamNames=[]  SerializedMaskParamValues=[]  SerializedMaskParamVisibilities=[]  block_type=IDFT  SerializedMaskParamDataypes=typename|typename|uint|uint|uint|uint|uint|uint|uint|uint|uint|uint  SerializedMaskParamEnumStrArr=0|0|0|0|0|Floor,Ceiling,Round to positive infinity,Round to negative infinity,Round symmetrical to infinity,Round symmetrical to zero,Round convergent to even,Round convergent to odd|0|0-None,1-Asymmetric,3-Symmetric|0|0|0|0  SerializedMaskParamEnumValArr=0|0|0|0|0|0,1,2,3,4,5,6,7|0|0,1,3|0|0|0|0  SerializedMaskParamVectorArr=0|0|0|0|0|0|0|0|0|0|0|0  SerializedMaskParamKeys=TT_DATA|TT_TWIDDLE|TP_POINT_SIZE|TP_NUM_FRAMES|TP_SHIFT|TP_RND|TP_SSR|TP_SAT|TP_CASC_LEN|AIE_VARIANT|TP_API|TP_FFT_NIFFT
  IDFT_Half1 : aieDSP/IDFT  data_type=cint16  twiddle_type=cint16  point_size=16  num_frames=256  shift_val=0  rnd_mode=Round to positive infinity  ssr=4  sat_mode=1-Asymmetric  casc_length=4  AIE_VARIANT=1  TP_API=0  TP_FFT_NIFFT=0  blockJsonConstraints=[]  blockJsonConstraintsInternal=[]  spec=vmc_idft.json  SerializedMaskParamNames=[]  SerializedMaskParamValues=[]  SerializedMaskParamVisibilities=[]  block_type=IDFT  SerializedMaskParamDataypes=typename|typename|uint|uint|uint|uint|uint|uint|uint|uint|uint|uint  SerializedMaskParamEnumStrArr=0|0|0|0|0|Floor,Ceiling,Round to positive infinity,Round to negative infinity,Round symmetrical to infinity,Round symmetrical to zero,Round convergent to even,Round convergent to odd|0|0-None,1-Asymmetric,3-Symmetric|0|0|0|0  SerializedMaskParamEnumValArr=0|0|0|0|0|0,1,2,3,4,5,6,7|0|0,1,3|0|0|0|0  SerializedMaskParamVectorArr=0|0|0|0|0|0|0|0|0|0|0|0  SerializedMaskParamKeys=TT_DATA|TT_TWIDDLE|TP_POINT_SIZE|TP_NUM_FRAMES|TP_SHIFT|TP_RND|TP_SSR|TP_SAT|TP_CASC_LEN|AIE_VARIANT|TP_API|TP_FFT_NIFFT
  MergeHalf0 : aieUtilities/Merger  ssr=4  PreSSR=4
  MergeHalf1 : aieUtilities/Merger  ssr=4  PreSSR=4
  PLIO_In_Half0 : aieBasic/PLIO  PlioWidth=64  PlioFreqSpec=on  PlioFreq=625  ColLocation=0  channel=0  blockJsonConstraints=[]  deprecateConstraints=0
  PLIO_In_Half1 : aieBasic/PLIO  PlioWidth=64  PlioFreqSpec=on  PlioFreq=625  ColLocation=0  channel=0  blockJsonConstraints=[]  deprecateConstraints=0
  PLIO_Out_Half0 : aieBasic/PLIO  PlioWidth=64  PlioFreqSpec=on  PlioFreq=625  ColLocation=0  channel=0  blockJsonConstraints=[]  deprecateConstraints=0
  PLIO_Out_Half1 : aieBasic/PLIO  PlioWidth=64  PlioFreqSpec=on  PlioFreq=625  ColLocation=0  channel=0  blockJsonConstraints=[]  deprecateConstraints=0
  SplitHalf0 : aieUtilities/Splitter  ssr=16  PreSSR=16
  SplitHalf1 : aieUtilities/Splitter  ssr=16  PreSSR=16
  IDFT_Half0_Out : Outport
  IDFT_Half1_Out : Outport  Port=2
  wires:
  PLIO_Out_Half0/1 -> IDFT_Half0_Out/1
  In_Half0/1 -> PLIO_In_Half0/1
  In_Half1/1 -> PLIO_In_Half1/1
  PLIO_In_Half0/1 -> SplitHalf0/1
  PLIO_In_Half1/1 -> SplitHalf1/1
  MergeHalf1/1 -> PLIO_Out_Half1/1
  PLIO_Out_Half1/1 -> IDFT_Half1_Out/1
  MergeHalf0/1 -> PLIO_Out_Half0/1
  SplitHalf0/1 -> IDFT_Half0/1
  SplitHalf0/2 -> IDFT_Half0/2
  SplitHalf0/3 -> IDFT_Half0/3
  SplitHalf0/4 -> IDFT_Half0/4
  SplitHalf0/5 -> IDFT_Half0/5
  SplitHalf0/6 -> IDFT_Half0/6
  SplitHalf0/7 -> IDFT_Half0/7
  SplitHalf0/8 -> IDFT_Half0/8
  SplitHalf0/9 -> IDFT_Half0/9
  SplitHalf0/10 -> IDFT_Half0/10
  SplitHalf0/11 -> IDFT_Half0/11
  SplitHalf0/12 -> IDFT_Half0/12
  SplitHalf0/13 -> IDFT_Half0/13
  SplitHalf0/14 -> IDFT_Half0/14
  SplitHalf0/15 -> IDFT_Half0/15
  SplitHalf0/16 -> IDFT_Half0/16
  IDFT_Half0/1 -> MergeHalf0/1
  IDFT_Half0/2 -> MergeHalf0/2
  IDFT_Half0/3 -> MergeHalf0/3
  IDFT_Half0/4 -> MergeHalf0/4
  SplitHalf1/1 -> IDFT_Half1/1
  SplitHalf1/2 -> IDFT_Half1/2
  SplitHalf1/3 -> IDFT_Half1/3
  SplitHalf1/4 -> IDFT_Half1/4
  SplitHalf1/5 -> IDFT_Half1/5
  SplitHalf1/6 -> IDFT_Half1/6
  SplitHalf1/7 -> IDFT_Half1/7
  SplitHalf1/8 -> IDFT_Half1/8
  SplitHalf1/9 -> IDFT_Half1/9
  SplitHalf1/10 -> IDFT_Half1/10
  SplitHalf1/11 -> IDFT_Half1/11
  SplitHalf1/12 -> IDFT_Half1/12
  SplitHalf1/13 -> IDFT_Half1/13
  SplitHalf1/14 -> IDFT_Half1/14
  SplitHalf1/15 -> IDFT_Half1/15
  SplitHalf1/16 -> IDFT_Half1/16
  IDFT_Half1/1 -> MergeHalf1/1
  IDFT_Half1/2 -> MergeHalf1/2
  IDFT_Half1/3 -> MergeHalf1/3
  IDFT_Half1/4 -> MergeHalf1/4
